simulink library "uSimLib"  (Simulink 7.8)
settings: Solver=ode45  StartTime=0.0  StopTime=10.0  RelTol=1e-3
libraries: simulink x6, aerolibconvert2 x4
(part 1 of 3)
settings Model: Creator=bwmairs  LastModifiedBy=Bryant

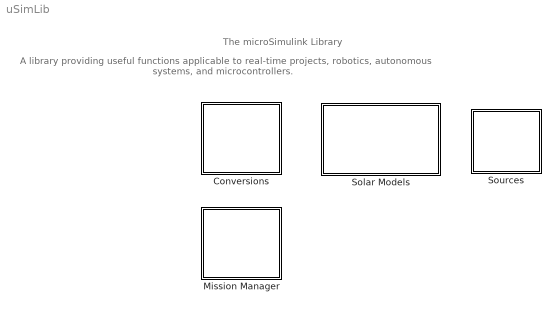
== system uSimLib ==
  note: The microSimulink Library
  note: A library providing useful functions applicable to real-time projects,
      | robotics, autonomous systems, and microcontrollers.
  Conversions : Subsystem
      mask Display: fprintf('A <-> B');
  Mission Manager : Subsystem
      mask Display: fprintf('Missions');
  Solar Models : Subsystem
      mask Display: fprintf('\\ | /\n- O -\n/ | \\');
  Sources : Subsystem
      mask Display: fprintf('^\n|');

== system uSimLib/Conversions ==
  Angle Conversion : Subsystem  mask(Angle Conversion){iu=rad, ou=deg}
      mask prompts: iu "Initial units:"; ou "Final units:"
      mask help: Convert units of rotation.
      mask init:
      | slope = 0;
      | if iu == 'deg'
      |     if ou == 'rad'
      |         slope = pi/180;
      |     elseif ou == 'rev'
      |         slope = 1/360;
      |     end
      | elseif iu == 'rad'
      |     if ou == 'deg'
      |         slope = 180/pi;
      |     elseif ou == 'rev'
      |         slope = 1/(2*pi);
      |     end
      | elseif iu == 'rev'
      |     if ou == 'deg'
      |         slope = 360;
      |     elseif ou == 'rad'
      |         slope = 2*pi;
      |     end
      | end
      mask StyleString: popup(deg|rad|rev),popup(deg|rad|rev)
      mask Display:
      | port_label('input', 1, get_param(gcb, 'iu'));
      | port_label('output', 1, get_param(gcb, 'ou'));
  uint16 to uchar : Subsystem
  uint32 to uchar : Subsystem

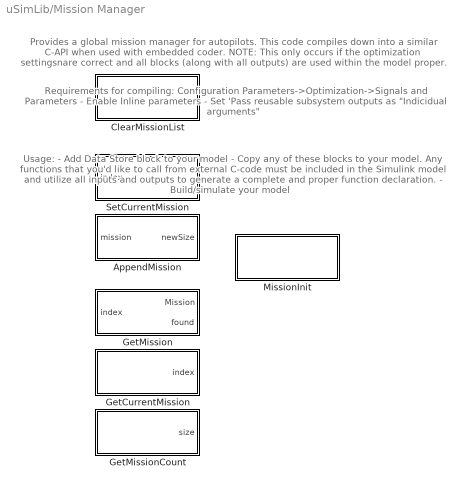
== system uSimLib/Mission Manager ==
  note: Provides a global mission manager for autopilots. This code compiles down
      | into a similar C-API when used with embedded coder. NOTE: This only occurs
      | if the optimization settingsnare correct and all blocks (along with all outputs)
      | are used within the model proper.
  note: Requirements for compiling:
      | Configuration Parameters->Optimization->Signals and Parameters
      |  - Enable Inline parameters
      |  - Set 'Pass reusable subsystem outputs as "Indicidual arguments"
  note: Usage:
      |  - Add Data Store block to your model
      |  - Copy any of these blocks to your model. Any functions that you'd like to call from external
      | C-code must be included in the Simulink model and utilize all inputs and outputs to generate
      | a complete and proper function declaration.
      |  - Build/simulate your model
  AppendMission : Subsystem  TreatAsAtomicUnit=on  RTWFcnName=AppendMission  RTWFileName=MissionManager  mask{sampleTime=-1}
      mask prompts: sampleTime "Sample time"
      settings: RTWFcnNameOpts=User specified  RTWFileNameOpts=User specified
  ClearMissionList : Subsystem  TreatAsAtomicUnit=on  RTWFcnName=ClearMissionList  RTWFileName=MissionManager  mask{sampleTime=-1}
      mask prompts: sampleTime "Sample time"
      settings: RTWFcnNameOpts=User specified  RTWFileNameOpts=User specified
      mask Display: disp('Mission:Clear()');
  GetCurrentMission : Subsystem  TreatAsAtomicUnit=on  RTWFcnName=GetCurrentMission  RTWFileName=MissionManager  mask{sampleTime=-1}
      mask prompts: sampleTime "Sample time"
      settings: RTWFcnNameOpts=User specified  RTWFileNameOpts=User specified
  GetMission : Subsystem  TreatAsAtomicUnit=on  RTWFcnName=GetMission  RTWFileName=MissionManager  mask{sampleTime=-1}
      mask prompts: sampleTime "Sample time"
      settings: RTWFcnNameOpts=User specified  RTWFileNameOpts=User specified
  GetMissionCount : Subsystem  TreatAsAtomicUnit=on  RTWFcnName=GetMissionCount  RTWFileName=MissionManager  mask{sampleTime=-1}
      mask prompts: sampleTime "Sample time"
      settings: RTWFcnNameOpts=User specified  RTWFileNameOpts=User specified
  MissionInit : Subsystem  LoadFcn=|  InitFcn=|  TreatAsAtomicUnit=on  RTWFcnName=MissionInit  RTWFileName=MissionManager
      LoadFcn=|
      | % Bus object: Mission                                                                                                                                                                           
      | clear elems;                                                                                                                                                                                    
      | elems(1) = Simulink.BusElement;                                                                                                                                                                 
      | elems(1).Name = 'coordinates';                                                                                                                                                                  
      | elems(1).Dimensions = 3;                                                                                                                                                                        
      | elems(1).DimensionsMode = 'Fixed';                                                                                                                                                              
      | elems(1).DataType = 'single';                                                                                                                                                                   
      | elems(1).SampleTime = -1;                                                                                                                                                                       
      | elems(1).Complexity = 'real';                                                                                                                                                                   
      | elems(1).SamplingMode = 'Sample based';                                                                                                                                                         
      | elems(1).Min = [];                                                                                                                                                                              
      | elems(1).Max = [];                                                                                                                                                                              
      |                                                                                                                                                                                                 
      | elems(2) = Simulink.BusElement;                                                                                                                                                                 
      | elems(2).Name = 'refFrame';                                                                                                                                                                     
      | elems(2).Dimensions = 1;                                                                                                                                                                        
      | elems(2).DimensionsMode = 'Fixed';                                                                                                                                                              
      | elems(2).DataType = 'uint8';                                                                                                                                                                    
      | elems(2).SampleTime = -1;                                                                                                                                                                       
      | elems(2).Complexity = 'real';                                                                                                                                                                   
      | elems(2).SamplingMode = 'Sample based';                                                                                                                                                         
      | elems(2).Min = [];                                                                                                                                                                              
      | elems(2).Max = [];                                                                                                                                                                              
      |                                                                                                                                                                                                 
      | elems(3) = Simulink.BusElement;                                                                                                                                                                 
      | elems(3).Name = 'action';                                                                                                                                                                       
      | elems(3).Dimensions = 1;                                                                                                                                                                        
      | elems(3).DimensionsMode = 'Fixed';                                                                                                                                                              
      | elems(3).DataType = 'uint8';                                                                                                                                                                    
      | elems(3).SampleTime = -1;                                                                                                                                                                       
      | elems(3).Complexity = 'real';                                                                                                                                                                   
      | elems(3).SamplingMode = 'Sample based';                                                                                                                                                         
      | elems(3).Min = [];                                                                                                                                                                              
      | elems(3).Max = [];                                                                                                                                                                              
      |                                                                                                                                                                                                 
      | elems(4) = Simulink.BusElement;                                                                                                                                                                 
      | elems(4).Name = 'parameters';                                                                                                                                                                   
      | elems(4).Dimensions = 4;                                                                                                                                                                        
      | elems(4).DimensionsMode = 'Fixed';                                                                                                                                                              
      | elems(4).DataType = 'single';                                                                                                                                                                   
      | elems(4).SampleTime = -1;                                                                                                                                                                       
      | elems(4).Complexity = 'real';                                                                                                                                                                   
      | elems(4).SamplingMode = 'Sample based';                                                                                                                                                         
      | elems(4).Min = [];                                                                                                                                                                              
      | elems(4).Max = [];                                                                                                                                                                              
      |                                                                                                                                                                                                 
      | elems(5) = Simulink.BusElement;                                                                                                                                                                 
      | elems(5).Name = 'autocontinue';                                                                                                                                                                 
      | elems(5).Dimensions = 1;                                                                                                                                                                        
      | elems(5).DimensionsMode = 'Fixed';                                                                                                                                                              
      | elems(5).DataType = 'boolean';                                                                                                                                                                  
      | elems(5).SampleTime = -1;                                                                                                                                                                       
      | elems(5).Complexity = 'real';                                                                                                                                                                   
      | elems(5).SamplingMode = 'Sample based';                                                                                                                                                         
      | elems(5).Min = [];                                                                                                                                                                              
      | elems(5).Max = [];                                                                                                                                                                              
      |                                                                                                                                                                                                 
      | Mission = Simulink.Bus;                                                                                                                                                                         
      | Mission.HeaderFile = '';                                                                                                                                                                        
      | Mission.Description = sprintf('Contains all of the parameters necessary for fully defining missions (aka waypoints) for the autopilot. Follows directly from how MAVLink implements missions.');
      | Mission.DataScope = 'Auto';                                                                                                                                                                     
      | Mission.Alignment = -1;                                                                                                                                                                         
      | Mission.Elements = elems;                                                                                                                                                                       
      | assignin('base', 'Mission', Mission)                                                                                                                                                            
      |                                                                                                                                                                                                 
      | % Bus object: MissionList                                                                                                                                                                       
      | clear elems;                                                                                                                                                                                    
      | elems(1) = Simulink.BusElement;                                                                                                                                                                 
      | elems(1).Name = 'currentIndex';                                                                                                                                                                 
      | elems(1).Dimensions = 1;                                                                                                                                                                        
      | elems(1).DimensionsMode = 'Fixed';                                                                                                                                                              
      | elems(1).DataType = 'uint8';                                                                                                                                                                    
      | elems(1).SampleTime = -1;                                                                                                                                                                       
      | elems(1).Complexity = 'real';                                                                                                                                                                   
      | elems(1).SamplingMode = 'Sample based';                                                                                                                                                         
      | elems(1).Min = [];                                                                                                                                                                              
      | elems(1).Max = [];                                                                                                                                                                              
      |                                                                                                                                                                                                 
      | elems(2) = Simulink.BusElement;                                                                                                                                                                 
      | elems(2).Name = 'size';                                                                                                                                                                         
      | elems(2).Dimensions = 1;                                                                                                                                                                        
      | elems(2).DimensionsMode = 'Fixed';                                                                                                                                                              
      | elems(2).DataType = 'uint8';                                                                                                                                                                    
      | elems(2).SampleTime = -1;                                                                                                                                                                       
      | elems(2).Complexity = 'real';                                                                                                                                                                   
      | elems(2).SamplingMode = 'Sample based';                                                                                                                                                         
      | elems(2).Min = [];                                                                                                                                                                              
      | elems(2).Max = [];                                                                                                                                                                              
      |                                                                                                                                                                                                 
      | elems(3) = Simulink.BusElement;                                                                                                                                                                 
      | elems(3).Name = 'missions';                                                                                                                                                                     
      | elems(3).Dimensions = 15;                                                                                                                                                                       
      | elems(3).DimensionsMode = 'Fixed';                                                                                                                                                              
      | elems(3).DataType = 'Bus: Mission';                                                                                                                                                             
      | elems(3).SampleTime = -1;                                                                                                                                                                       
      | elems(3).Complexity = 'real';                                                                                                                                                                   
      | elems(3).SamplingMode = 'Sample based';                                                                                                                                                         
      | elems(3).Min = [];                                                                                                                                                                              
      | elems(3).Max = [];                                                                                                                                                                              
      |                                                                                                                                                                                                 
      | MissionList = Simulink.Bus;                                                                                                                                                                     
      | MissionList.HeaderFile = '';                                                                                                                                                                    
      | MissionList.Description = sprintf('This is the central data store for the various Missions that will be used by the autopilot.');                                                               
      | MissionList.DataScope = 'Auto';                                                                                                                                                                 
      | MissionList.Alignment = -1;                                                                                                                                                                     
      | MissionList.Elements = elems;                                                                                                                                                                   
      | assignin('base', 'MissionList', MissionList)
      InitFcn=|
      | mList = Simulink.Signal;
      | mList.RTWInfo.StorageClass = 'ExportedGlobal';
      | mList.RTWInfo.Alias = '';
      | mList.RTWInfo.Alignment = -1;
      | mList.RTWInfo.CustomStorageClass = 'Default';
      | mList.Description = '';
      | mList.DataType = 'Bus: MissionList';
      | mList.Min = [];
      | mList.Max = [];
      | mList.DocUnits = '';
      | mList.Dimensions = 1;
      | mList.DimensionsMode = 'auto';
      | mList.Complexity = 'real';
      | mList.SampleTime = -1;
      | mList.SamplingMode = 'Sample based';
      | mList.InitialValue = '';
      | assignin('base', 'mList', mList);
      settings: RTWFcnNameOpts=User specified  RTWFileNameOpts=User specified
      mask Description: Initialization block for the Mission Manager.
      mask Display: disp('Mission: Init()');
  SetCurrentMission : Subsystem  TreatAsAtomicUnit=on  RTWFcnName=SetCurrentMission  RTWFileName=MissionManager  mask{sampleTime=-1}
      mask prompts: sampleTime "Sample time"
      settings: RTWFcnNameOpts=User specified  RTWFileNameOpts=User specified

== system uSimLib/Solar Models ==
  Embedded MATLAB Function : MATLAB Function  TreatAsAtomicUnit=on
  Solar Position (in translation) : Subsystem

== system uSimLib/Sources ==
  Discrete step : Subsystem  mask(Discrete step){start_value=1, end_value=0, transition_time=500}
      mask prompts: start_value "Initial value"; end_value "Final value"; transition_time "Transition time"
      mask help:
      | This block implements a single-transition step output. Transition time is
      | the timestep at which this block should change its output value in the
      | units of the base timestep.
      mask Display:
      | X = [0 0.5 0.5 1];
      | 
      | if (start_value < end_value)
      |     Y = [0 0 1 1];
      | else
      |     Y = [1 1 0 0];
      | end
      | 
      | plot(X,Y)

== system uSimLib/Conversions/Angle Conversion ==
  In1 : Inport
  Gain : Gain  Gain=slope
  Out1 : Outport
  wires:
  Gain/1 -> Out1/1
  In1/1 -> Gain/1

== system uSimLib/Conversions/uint16 to uchar ==
  ushort : Inport
  Data Type Conversion : DataTypeConversion  OutDataTypeStr=uint16  ConvertRealWorld=Stored Integer (SI)  RndMeth=Simplest
  Extract Bits1 : simulink/Logic and Bit Operations/Extract Bits  bitsToExtract=Lower half  numBits=8  bitIdxRange=[0 7]  outScalingMode=Treat bit field as an integer
  Extract Bits2 : simulink/Logic and Bit Operations/Extract Bits  bitsToExtract=Upper half  numBits=8  bitIdxRange=[0 7]  outScalingMode=Treat bit field as an integer
  Mux : Mux  Inputs=2
  uchar : Outport
  wires:
  Mux/1 -> uchar/1
  Extract Bits2/1 -> Mux/2
  Extract Bits1/1 -> Mux/1
  ushort/1 -> Data Type Conversion/1
  Data Type Conversion/1 -> Extract Bits1/1, Extract Bits2/1

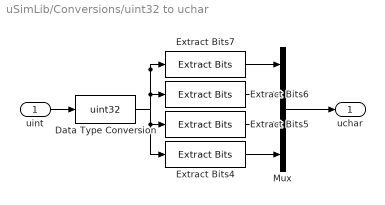
== system uSimLib/Conversions/uint32 to uchar ==
  uint : Inport
  Data Type Conversion : DataTypeConversion  OutDataTypeStr=uint32  ConvertRealWorld=Stored Integer (SI)  RndMeth=Simplest
  Extract Bits4 : simulink/Logic and Bit Operations/Extract Bits  bitsToExtract=Range of bits  numBits=8  bitIdxRange=[24 31]  outScalingMode=Treat bit field as an integer
  Extract Bits5 : simulink/Logic and Bit Operations/Extract Bits  bitsToExtract=Range of bits  numBits=8  bitIdxRange=[16 23]  outScalingMode=Treat bit field as an integer
  Extract Bits6 : simulink/Logic and Bit Operations/Extract Bits  bitsToExtract=Range of bits  numBits=8  bitIdxRange=[8 15]  outScalingMode=Treat bit field as an integer
  Extract Bits7 : simulink/Logic and Bit Operations/Extract Bits  bitsToExtract=Range of bits  numBits=8  bitIdxRange=[0 7]  outScalingMode=Treat bit field as an integer
  Mux : Mux
  uchar : Outport
  wires:
  Data Type Conversion/1 -> Extract Bits7/1, Extract Bits6/1, Extract Bits5/1, Extract Bits4/1
  Extract Bits4/1 -> Mux/4
  Extract Bits5/1 -> Mux/3
  Extract Bits6/1 -> Mux/2
  Extract Bits7/1 -> Mux/1
  uint/1 -> Data Type Conversion/1
  Mux/1 -> uchar/1

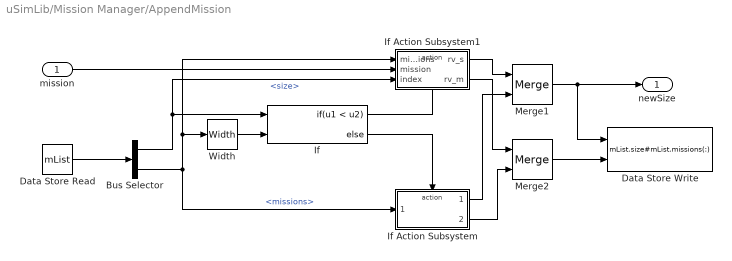
== system uSimLib/Mission Manager/AppendMission ==
  mission : Inport  OutDataTypeStr=Bus: Mission
  Bus Selector : BusSelector  OutputSignals=size,missions
  Data Store Read : DataStoreRead  DataStoreName=mList  SampleTime=sampleTime
  Data Store Write : DataStoreWrite  DataStoreName=mList  SampleTime=sampleTime  DataStoreElements=mList.size#mList.missions(:)
  If : If  NumInputs=2  IfExpression=u1 < u2  ZeroCross=off
  If Action Subsystem : Subsystem  TreatAsAtomicUnit=on
  If Action Subsystem1 : Subsystem  TreatAsAtomicUnit=on
  Merge1 : Merge
  Merge2 : Merge
  Width : Width  DataType=uint8
  newSize : Outport  OutDataTypeStr=uint8  LockScale=on
  wires:
  If Action Subsystem1/1(rv_s) -> Merge1/1
  If Action Subsystem/1(rv_found) -> Merge1/2
  Merge1/1 -> newSize/1, Data Store Write/1
  If/1 -> If Action Subsystem1/Action
  Bus Selector/2 -> If Action Subsystem/1(missions), Width/1, If Action Subsystem1/1(missions)  "<missions>"
  If/2 -> If Action Subsystem/Action
  Width/1 -> If/2
  Data Store Read/1 -> Bus Selector/1
  mission/1 -> If Action Subsystem1/2(mission)
  If Action Subsystem1/2(rv_m) -> Merge2/1
  If Action Subsystem/2(rv_missions) -> Merge2/2
  Merge2/1 -> Data Store Write/2
  Bus Selector/1 -> If Action Subsystem1/3(index), If/1  "<size>"

== system uSimLib/Mission Manager/ClearMissionList ==
  Constant : Constant  Value=0  OutDataTypeStr=uint8
  Data Store Write : DataStoreWrite  DataStoreName=mList  SampleTime=sampleTime  DataStoreElements=mList.size
  wires:
  Constant/1 -> Data Store Write/1

== system uSimLib/Mission Manager/GetCurrentMission ==
  Data Store Read1 : DataStoreRead  DataStoreName=mList  SampleTime=sampleTime  DataStoreElements=mList.currentIndex
  index : Outport  OutDataTypeStr=uint8
  wires:
  Data Store Read1/1 -> index/1

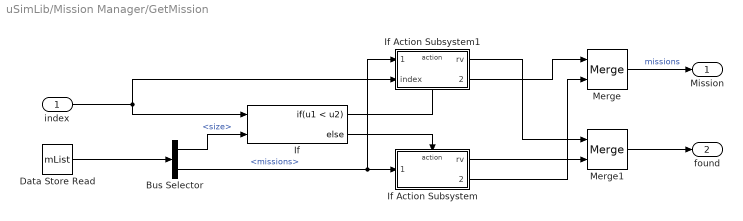
== system uSimLib/Mission Manager/GetMission ==
  index : Inport  OutDataTypeStr=uint8
  Bus Selector : BusSelector  OutputSignals=size,missions
  Data Store Read : DataStoreRead  DataStoreName=mList  SampleTime=sampleTime
  If : If  NumInputs=2  IfExpression=u1 < u2
  If Action Subsystem : Subsystem  TreatAsAtomicUnit=on
  If Action Subsystem1 : Subsystem  TreatAsAtomicUnit=on
  Merge : Merge
  Merge1 : Merge
  Mission : Outport  OutDataTypeStr=Bus: Mission
  found : Outport  Port=2  OutDataTypeStr=boolean
  wires:
  Data Store Read/1 -> Bus Selector/1
  Bus Selector/1 -> If/2  "<size>"
  index/1 -> If/1, If Action Subsystem1/2(index)
  Merge/1 -> Mission/1  "missions"
  If/2 -> If Action Subsystem/Action
  Bus Selector/2 -> If Action Subsystem1/1(missions), If Action Subsystem/1(missions)  "<missions>"
  If/1 -> If Action Subsystem1/Action
  Merge1/1 -> found/1
  If Action Subsystem/1(rv) -> Merge1/2
  If Action Subsystem1/1(rv) -> Merge1/1
  If Action Subsystem1/2(mission) -> Merge/1
  If Action Subsystem/2(mission) -> Merge/2

== system uSimLib/Mission Manager/GetMissionCount ==
  Data Store Read : DataStoreRead  DataStoreName=mList  SampleTime=sampleTime  DataStoreElements=mList.size
  size : Outport  OutDataTypeStr=uint8
  wires:
  Data Store Read/1 -> size/1

== system uSimLib/Mission Manager/MissionInit ==

== system uSimLib/Mission Manager/SetCurrentMission ==
  index : Inport  OutDataTypeStr=uint8
  Data Store Read : DataStoreRead  DataStoreName=mList  SampleTime=sampleTime  DataStoreElements=mList.size
  If : If  NumInputs=2  IfExpression=u1 < u2  ShowElse=off  ZeroCross=off
  If Action Subsystem : Subsystem  TreatAsAtomicUnit=on
  wires:
  index/1 -> If/1, If Action Subsystem/1(In1)
  Data Store Read/1 -> If/2
  If/1 -> If Action Subsystem/Action

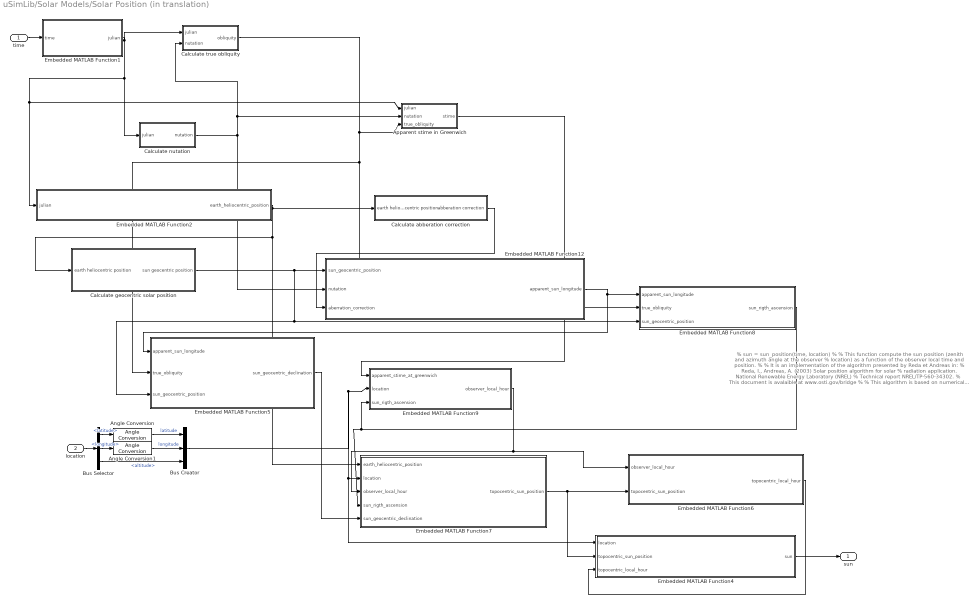
== system uSimLib/Solar Models/Solar Position (in translation) ==
  note: % sun = sun_position(time, location)
      | %
      | % This function compute the sun position (zenith and azimuth angle at the observer
      | % location) as a function of the observer local time and position.
      | %
      | % It is an implementation of the algorithm presented by Reda et Andreas in:
      | %   Reda, I., Andreas, A. (2003) Solar position algorithm for solar
      | %   radiation application. National Renewable Energy Laboratory (NREL)
      | %   Technical report NREL/TP-560-34302.
      | % This document is avalaible at www.osti.gov/bridge
      | %
      | % This algorithm is based on numerical approximation of the exact equations.
      | % The authors of the original paper state that this algorithm should be
      | % precise at +/- 0.0003 degrees. I have compared it to NOAA solar table
      | % (http://www.srrb.noaa.gov/highlights/sunrise/azel.html) and to USNO solar
      | % table (http://aa.usno.navy.mil/data/docs/AltAz.html) and found very good
      | % correspondance (up to the precision of those tables), except for large
      | % zenith angle, where the refraction by the atmosphere is significant
      | % (difference of about 1 degree). Note that in this code the correction
      | % for refraction in the atmosphere as been implemented for a temperature
      | % of 10C (283 kelvins) and a pressure of 1010 mbar. See the subfunction
      | % «sun_topocentric_zenith_angle_calculation» for a possible modification
      | % to explicitely model the effect of temperature and pressure as describe
      | % in Reda & Andreas (2003).
      | %
      | % Input parameters:
      | %   time: a structure that specify the time when the sun position is
      | %   calculated.
      | %       time.year: year. Valid for [-2000, 6000]
      | %       time.month: month [1-12]
      | %       time.day: calendar day [1-31]
      | %       time.hour: local hour [0-23]
      | %       time.min: minute [0-59]
      | %       time.sec: second [0-59]
      | %       time.UTC: offset hour from UTC. Local time = Greenwich time + time.UTC
      | %   This input can also be passed using the Matlab time format ('dd-mmm-yyyy HH:MM:SS').
      | %   In that case, the time has to be specified as UTC time (time.UTC = 0)
      | %
      | %   location: a structure that specify the location of the observer
      | %       location.latitude: latitude (in degrees, north of equator is
      | %       positive)
      | %       location.longitude: longitude (in degrees, positive for east of
      | %       Greenwich)
      | %       location.altitude: altitude above mean sea level (in meters)
      | %
      | % Output parameters
      | %   sun: a structure with the calculated sun position
      | %       sun.zenith = zenith angle in degrees (angle from the vertical)
      | %       sun.azimuth = azimuth angle in degrees, eastward from the north.
      | % Only the sun zenith and azimuth angles are returned as output, but a lot
      | % of other parameters are calculated that could also extracted as output of
      | % this function.
      | %
      | % Exemple of use
      | %
      | % location.longitude = -105.1786;
      | % location.latitude = 39.742476;
      | % location.altitude = 1830.14;
      | % time.year = 2003;
      | % time.month = 10;
      | % time.day = 17;
      | % time.hour = 12;
      | % time.min = 30;
      | % time.sec = 30;
      | % time.UTC = -7;
      | %
      | % sun = sun_position(time, location);
      | %
      | % sun =
      | %
      | %      zenith: 50.1080438859849
      | %      azimuth: 194.341174010338
      | %
      | % History
      | %   09/03/2004  Original creation by Vincent Roy (vincent.roy@drdc-rddc.gc.ca)
      | %   10/03/2004  Fixed a bug in julian_calculation subfunction (was
      | %               incorrect for year 1582 only), Vincent Roy
      | %   18/03/2004  Correction to the header (help display) only. No changes to
      | %               the code. (changed the «elevation» field in «location» structure
      | %               information to «altitude»), Vincent Roy
      | %   13/04/2004  Following a suggestion from Jody Klymak (jklymak@ucsd.edu),
      | %               allowed the 'time' input to be passed as a Matlab time string.
      | %   22/08/2005  Following a bug report from Bruce Bowler
      | %               (bbowler@bigelow.org), modified the julian_calculation function. Bug
      | %               was 'MATLAB has allowed structure assignment  to a non-empty non-structure
      | %               to overwrite the previous value.  This behavior will continue in this release,
      | %               but will be an error in a  future version of MATLAB.  For advice on how to
      | %               write code that  will both avoid this warning and work in future versions of
      | %               MATLAB,  see R14SP2 Release Notes'. Script should now be
      | %               compliant with futher release of Matlab...
  time : Inport
  location : Inport  Port=2
  Angle Conversion : aerolibconvert2/Angle Conversion  IU=rad  OU=deg
  Angle Conversion1 : aerolibconvert2/Angle Conversion  IU=rad  OU=deg
  Apparent stime in Greenwich : Subsystem
  Bus Creator : BusCreator  Inputs=3  OutDataTypeStr=Bus: Location  NonVirtualBus=on
  Bus Selector : BusSelector  OutputSignals=latitude,longitude,altitude
  Calculate nutation : Subsystem
  Calculate abberation correction : Subsystem
  Calculate geocentric solar position : Subsystem
  Calculate true obliquity : Subsystem
  Embedded MATLAB Function1 : MATLAB Function  TreatAsAtomicUnit=on
  Embedded MATLAB Function12 : MATLAB Function  TreatAsAtomicUnit=on
  Embedded MATLAB Function2 : MATLAB Function  TreatAsAtomicUnit=on
  Embedded MATLAB Function4 : MATLAB Function  TreatAsAtomicUnit=on
  Embedded MATLAB Function5 : MATLAB Function  TreatAsAtomicUnit=on
  Embedded MATLAB Function6 : MATLAB Function  TreatAsAtomicUnit=on
  Embedded MATLAB Function7 : MATLAB Function  TreatAsAtomicUnit=on
  Embedded MATLAB Function8 : MATLAB Function  TreatAsAtomicUnit=on
  Embedded MATLAB Function9 : MATLAB Function  TreatAsAtomicUnit=on
  sun : Outport
  wires:
  Bus Selector/3 -> Bus Creator/3  "<altitude>"
  Bus Creator/1 -> Embedded MATLAB Function4/1(location), Embedded MATLAB Function7/2(location), Embedded MATLAB Function9/2(location)
  Angle Conversion1/1 -> Bus Creator/2  "longitude"
  Bus Selector/2 -> Angle Conversion1/1  "<longitude>"
  Angle Conversion/1 -> Bus Creator/1  "latitude"
  Bus Selector/1 -> Angle Conversion/1  "<latitude>"
  location/1 -> Bus Selector/1
  Embedded MATLAB Function4/1(sun) -> sun/1
  Embedded MATLAB Function6/1(topocentric_local_hour) -> Embedded MATLAB Function4/3(topocentric_local_hour)
  Embedded MATLAB Function7/1(topocentric_sun_position) -> Embedded MATLAB Function4/2(topocentric_sun_position), Embedded MATLAB Function6/2(topocentric_sun_position)
  Embedded MATLAB Function9/1(observer_local_hour) -> Embedded MATLAB Function6/1(observer_local_hour), Embedded MATLAB Function7/3(observer_local_hour)
  Embedded MATLAB Function5/1(sun_geocentric_declination) -> Embedded MATLAB Function7/5(sun_geocentric_declination)
  Apparent stime in Greenwich/1(stime) -> Embedded MATLAB Function9/1(apparent_stime_at_greenwich)
  Embedded MATLAB Function8/1(sun_rigth_ascension) -> Embedded MATLAB Function7/4(sun_rigth_ascension), Embedded MATLAB Function9/3(sun_rigth_ascension)
  Embedded MATLAB Function12/1(apparent_sun_longitude) -> Embedded MATLAB Function5/1(apparent_sun_longitude), Embedded MATLAB Function8/1(apparent_sun_longitude)
  Calculate true obliquity/1(obliquity) -> Embedded MATLAB Function8/2(true_obliquity), Embedded MATLAB Function5/2(true_obliquity), Apparent stime in Greenwich/3(true_obliquity)
  Calculate abberation correction/1(abberation correction) -> Embedded MATLAB Function12/3(aberration_correction)
  Calculate geocentric solar position/1(sun geocentric position) -> Embedded MATLAB Function5/3(sun_geocentric_position), Embedded MATLAB Function8/3(sun_geocentric_position), Embedded MATLAB Function12/1(sun_geocentric_position)
  Calculate nutation/1(nutation) -> Calculate true obliquity/2(nutation), Apparent stime in Greenwich/2(nutation), Embedded MATLAB Function12/2(nutation)
  Embedded MATLAB Function2/1(earth_heliocentric_position) -> Embedded MATLAB Function7/1(earth_heliocentric_position), Calculate geocentric solar position/1(earth heliocentric position), Calculate abberation correction/1(earth heliocentric position)
  Embedded MATLAB Function1/1(julian) -> Embedded MATLAB Function2/1(julian), Apparent stime in Greenwich/1(julian), Calculate nutation/1(julian), Calculate true obliquity/1(julian)
  time/1 -> Embedded MATLAB Function1/1(time)

== system uSimLib/Sources/Discrete step ==
  Constant : Constant  Value=start_value  OutDataTypeStr=uint8
  Constant1 : Constant  Value=end_value  OutDataTypeStr=uint8
  Constant2 : Constant  Value=transition_time  OutDataTypeStr=uint16
  Embedded MATLAB Function : MATLAB Function  TreatAsAtomicUnit=on
  Out1 : Outport
  wires:
  Embedded MATLAB Function/1(y) -> Out1/1
  Constant/1 -> Embedded MATLAB Function/1(start_value)
  Constant1/1 -> Embedded MATLAB Function/2(end_value)
  Constant2/1 -> Embedded MATLAB Function/3(transition_time)

== system uSimLib/Mission Manager/AppendMission/If Action Subsystem ==
  missions : Inport
  Action Port : ActionPort
  Constant : Constant  Value=0  OutDataTypeStr=uint8
  rv_found : Outport
  rv_missions : Outport  Port=2
  wires:
  Constant/1 -> rv_found/1
  missions/1 -> rv_missions/1

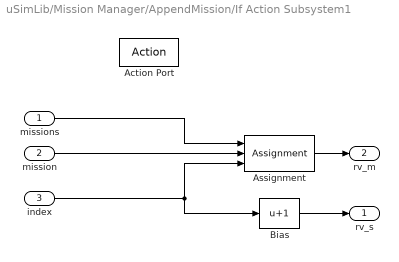
== system uSimLib/Mission Manager/AppendMission/If Action Subsystem1 ==
  missions : Inport
  mission : Inport  Port=2
  index : Inport  Port=3
  Action Port : ActionPort
  Assignment : Assignment  IndexMode=Zero-based  IndexOptions=Index vector (port)  Indices=1  OutputSizes=1
  Bias : Bias  Bias=1
  rv_s : Outport
  rv_m : Outport  Port=2
  wires:
  missions/1 -> Assignment/1
  mission/1 -> Assignment/2
  index/1 -> Assignment/3, Bias/1
  Assignment/1 -> rv_m/1
  Bias/1 -> rv_s/1

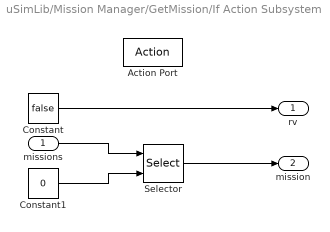
== system uSimLib/Mission Manager/GetMission/If Action Subsystem ==
  missions : Inport
  Action Port : ActionPort
  Constant : Constant  Value=false  OutDataTypeStr=boolean
  Constant1 : Constant  Value=0  OutDataTypeStr=uint8
  Selector : Selector  IndexMode=Zero-based  InputPortWidth=15  IndexOptions=Index vector (port)  Indices=[1 3]  OutputSizes=1
  rv : Outport
  mission : Outport  Port=2
  wires:
  Constant/1 -> rv/1
  Selector/1 -> mission/1
  Constant1/1 -> Selector/2
  missions/1 -> Selector/1

== system uSimLib/Mission Manager/GetMission/If Action Subsystem1 ==
  missions : Inport
  index : Inport  Port=2
  Action Port : ActionPort
  Constant : Constant  Value=true  OutDataTypeStr=boolean
  Selector : Selector  IndexMode=Zero-based  InputPortWidth=15  IndexOptions=Index vector (port)  Indices=[1 3]  OutputSizes=1
  rv : Outport
  mission : Outport  Port=2
  wires:
  Constant/1 -> rv/1
  Selector/1 -> mission/1
  index/1 -> Selector/2
  missions/1 -> Selector/1

== system uSimLib/Mission Manager/SetCurrentMission/If Action Subsystem ==
  In1 : Inport
  Action Port : ActionPort  ActionType=then
  Data Store Write : DataStoreWrite  DataStoreName=mList  SampleTime=sampleTime  DataStoreElements=mList.currentIndex
  wires:
  In1/1 -> Data Store Write/1

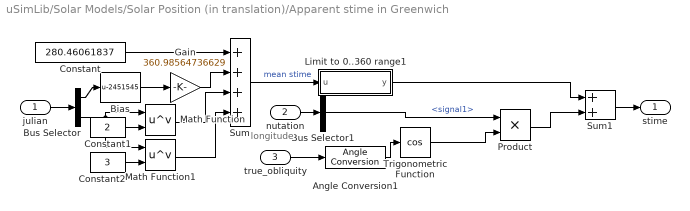
== system uSimLib/Solar Models/Solar Position (in translation)/Apparent stime in Greenwich ==
  note: longitude
  julian : Inport
  nutation : Inport  Port=2
  true_obliquity : Inport  Port=3
  Angle Conversion1 : aerolibconvert2/Angle Conversion  IU=deg  OU=rad
  Bias : Bias  Bias=-2451545
  Bus Selector : BusSelector  OutputSignals=signal1,signal2
  Bus Selector1 : BusSelector  OutputSignals=signal1
  Constant : Constant  Value=280.46061837
  Constant1 : Constant  Value=2
  Constant2 : Constant  Value=3
  Gain : Gain  Gain=360.98564736629
  Limit to 0..360 range1 : MATLAB Function  TreatAsAtomicUnit=on
  Math Function : Math  Operator=pow  SaturateOnIntegerOverflow=on
  Math Function1 : Math  Operator=pow  SaturateOnIntegerOverflow=on
  Product : Product  RndMeth=Zero
  Sum : Sum  Inputs=++++
  Sum1 : Sum
  Trigonometric Function : Trigonometry  Operator=cos
  stime : Outport
  wires:
  julian/1 -> Bus Selector/1
  Constant/1 -> Sum/1
  Bus Selector/1 -> Bias/1
  Bias/1 -> Gain/1
  Gain/1 -> Sum/2
  Bus Selector/2 -> Math Function/1, Math Function1/1
  Constant1/1 -> Math Function/2
  Math Function/1 -> Sum/3
  Constant2/1 -> Math Function1/2
  Math Function1/1 -> Sum/4
  Sum/1 -> Limit to 0..360 range1/1(u)  "mean stime"
  Limit to 0..360 range1/1(y) -> Sum1/1
  nutation/1 -> Bus Selector1/1
  true_obliquity/1 -> Angle Conversion1/1
  Angle Conversion1/1 -> Trigonometric Function/1
  Trigonometric Function/1 -> Product/2
  Product/1 -> Sum1/2
  Bus Selector1/1 -> Product/1  "<signal1>"
  Sum1/1 -> stime/1
